simulink subsystem "logica_obstaculos"  (R2023b)
settings: Solver=VariableStepAuto  StartTime=0.0  StopTime=10.0  RelTol=1e-3
libraries: simulink x2
settings Model: Creator=Manuel  LastModifiedBy=Usuario_UMA

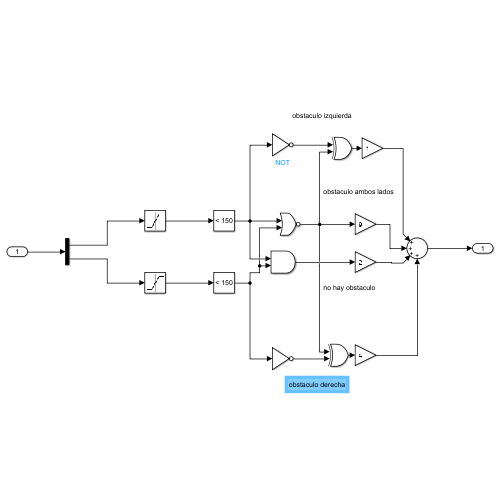
[thumbnail: Simulink's stored preview of the top-level diagram]
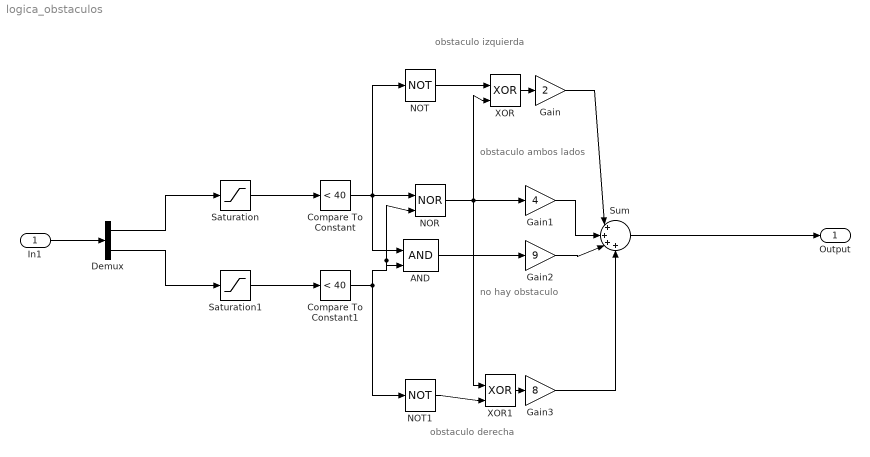
== system logica_obstaculos ==
  note: obstaculo ambos lados
  note: no hay obstaculo
  note: obstaculo derecha
  note: obstaculo izquierda
  In1 : Inport
  AND : Logic  IconShape=distinctive  AllPortsSameDT=off  OutDataTypeStr=boolean
  Compare To Constant : simulink/Logic and Bit Operations/Compare To Constant  relop=<  const=40  OutDataTypeStr=boolean
  Compare To Constant1 : simulink/Logic and Bit Operations/Compare To Constant  relop=<  const=40  OutDataTypeStr=boolean
  Demux : Demux  Outputs=2
  Gain : Gain  Gain=2
  Gain1 : Gain  Gain=4
  Gain2 : Gain  Gain=9
  Gain3 : Gain  Gain=8
  NOR : Logic  Operator=NOR  IconShape=distinctive  AllPortsSameDT=off  OutDataTypeStr=boolean
  NOT : Logic  Operator=NOT  IconShape=distinctive  AllPortsSameDT=off  OutDataTypeStr=boolean
  NOT1 : Logic  Operator=NOT  IconShape=distinctive  AllPortsSameDT=off  OutDataTypeStr=boolean
  Saturation : Saturate  UpperLimit=150  LowerLimit=0
  Saturation1 : Saturate  UpperLimit=150  LowerLimit=0
  Sum : Sum  Inputs=|++++
  XOR : Logic  Operator=XOR  IconShape=distinctive  AllPortsSameDT=off  OutDataTypeStr=boolean
  XOR1 : Logic  Operator=XOR  IconShape=distinctive  AllPortsSameDT=off  OutDataTypeStr=boolean
  Output : Outport
  wires:
  In1/1 -> Demux/1
  Demux/1 -> Saturation/1
  Demux/2 -> Saturation1/1
  Saturation/1 -> Compare To Constant/1
  Saturation1/1 -> Compare To Constant1/1
  Compare To Constant1/1 -> NOT1/1, NOR/2, AND/2
  Compare To Constant/1 -> AND/1, NOR/1, NOT/1
  AND/1 -> Gain2/1
  NOR/1 -> XOR/2, XOR1/1, Gain1/1
  Gain/1 -> Sum/1
  Gain1/1 -> Sum/2
  Gain2/1 -> Sum/3
  Gain3/1 -> Sum/4
  XOR/1 -> Gain/1
  NOT/1 -> XOR/1
  XOR1/1 -> Gain3/1
  NOT1/1 -> XOR1/2
  Sum/1 -> Output/1
